simulink model "cn_i_128w_2k_do_al_r301"  (Simulink 6.2)
settings: Solver=ode45  StartTime=0.0  StopTime=1000  RelTol=1e-3
libraries: xbsIndex_r3 x390, xps_library x17, ddc_library x4, reorder_library x3, fft_library x2, pfb_library x2, simulink x1, delay_lib x1
(part 1 of 3)
settings Model: LastModifiedBy=manley
settings DebuggingCC: SolverPrmCheckMsg=warning

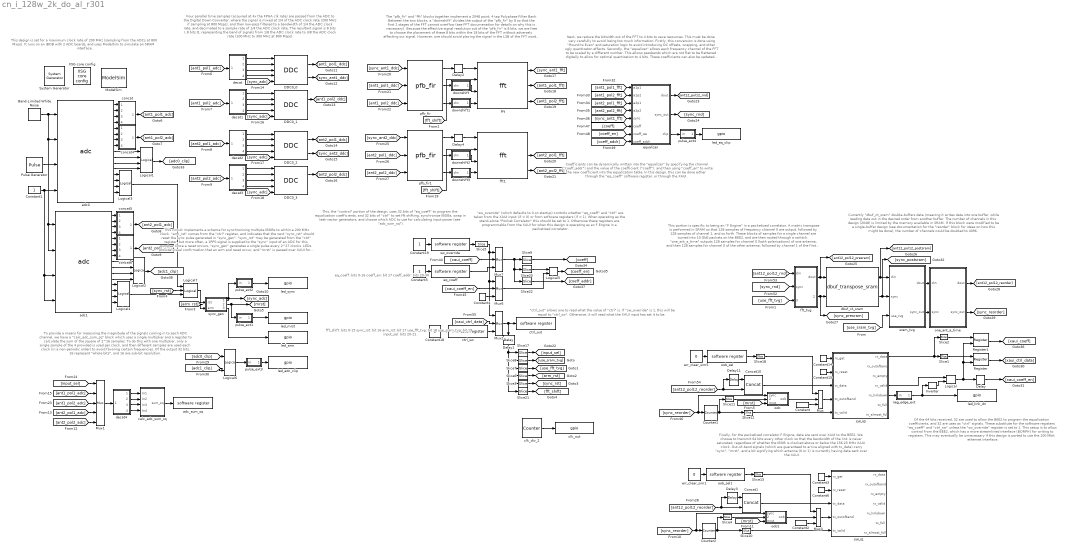
== system cn_i_128w_2k_do_al_r301 ==
  note: fft_shift: bits 0-15
      | sync_rst: bit 16
      | arm_rst: bit 17
      | use_fft_tvg: bit 18
      | use_sram_tvg: bit 19
      | input_sel: bits 20-21
  note: eq_coeff: bits 0-16
      | coeff_en: bit 17
      | coeff_addr: bits 20-30
  note: This design is set for a maximum
      | clock rate of 200 MHz (sampling
      | from the ADCs at 800 Mxps).  It
      | runs on an IBOB with 2 ADC boards,
      | and uses ModelSim to simulate an
      | SRAM interface.
  note: This circuit implements a scheme for synchronizing
      | multiple IBOBs to within a 200 MHz clock.  "arm_rst"
      | comes from the "ctrl" register, and indicates that the
      | next "sync_rst" should reset the sync pulse generated
      | in "sync_gen".  "sync_rst" may be generated from
      | the "ctrl" register, but more often, a 1PPS signal is
      | supplied to the "sync" input of an ADC for this
      | purpose.  Once a reset occurs, "sync_gen" generates
      | a single pulse every 2^27 clocks.  LEDs provide visual
      | confirmation that an arm and reset occur, and "mrst"
      | is passed over XAUI for the purpose of informing
      | downstream logic in a packetized correlator that
      | a "master reset" has occurred.
  note: "sw_override" (which defaults to 0 on startup)
      | controls whether "eq_coeff" and "ctrl" are taken
      | from the XAUI input (if = 0) or from software
      | registers (if = 1).  When operating as the stand-alone
      | "Pocket Correlator" this should be set to 1.  Otherwise
      | these registers are programmable from the XAUI for
      | when this design is operating as  an F Engine
      | in a packetized correlator.
  note: Four parallel time samples (acquired at 4x the
      | FPGA clk rate) are passed from the ADC to the
      | Digital Down Converter, where the signal is mixed
      | at 1/4 of the ADC clock rate (200 MHz if sampling
      | at 800 Msps), and then low-pass filtered to a
      | bandwidth of 1/4 the ADC clock rate, and decimated
      | to a sample rate of 1/4 the ADC clock rate.  The
      | resultant signal is 8 bits I, 8 bits Q, representing the
      | band of signals from 1/8 the ADC clock rate to
      | 3/8 the ADC clock rate (100 MHz to 300 MHz at
      | 800 Msps).
  note: The "pfb_fir" and "fft" blocks together implement a 2048 point,
      | 4 tap Polyphase Filter Bank.  Between the two blocks, a "downshift"
      | divides the output of the "pfb_fir" by 8 so that the first 2 stages of
      | the FFT cannot overflow (see FFT documenation for details on why
      | this is necessary).  Because the effective signal resolution out of
      | the "pfb_fir" is 8 bits, we are free to choose the placement of
      | these 8 bits within the 18 bits of the FFT without adversely affecting
      | our signal.  However, one should avoid placing the signal in the LSB
      | of the FFT word because of rounding effects.  Thus, we downshift
      | only 3 bits.
  note: Next, we reduce the bitwidth out of the FFT to 4 bits to save resources.
      | This must be done very carefully to avoid losing too much information.
      | Firstly, this conversion is done using "Round to Even" and saturation
      | logic to avoid introducing DC offsets, wrapping, and other ugly quantizaton
      | effects.  Secondly, the "equalizer" allows each frequency channel of the
      | FFT to be scaled by a different number.  This allows passbands which are
      | not flat to be flattened digitally to allow for optimal quantization to 4 bits.
      | These coefficients can also be updated dynamically for gain control.
  note: Coefficients can be dynamically written into the "equalizer" by
      | specifying the channel ("coeff_addr") and the value of the
      | coefficient ("coeff"), and then using "coeff_en" to write the
      | new coefficient into the equalization table.  In this design,
      | this can be done either through the "eq_coeff" software
      | register, or through the XAUI.
  note: To provide a means for measuring the magnitude of the signals
      | coming in to each ADC channel, we have a "calc_adc_sum_sq"
      | block which uses a single multiplier and a regsiter to calculate
      | the sum of the square of 2^16 samples.  To do this with one
      | multiplier, only a single sample of the 4 provided is used
      | per clock, and then different samples are used each clock (in
      | a non-periodic order) to avoid favoring certain frequencies.
      | Of the output 32 bits, 16 represent "whole bits", and 16
      | are sub-bit resolution.
  note: This portion is specific to being an "F Engine" in a packetized correlator.
      | A matrix transpose is performed in SRAM so that 128 samples of frequency
      | channel 0 are output, followed by 128 samples of channel 1, and so forth.
      | These blocks of samples for a single channel are turned into 10 GbE packets
      | on the BEE2, and are then routed through a swittch.  "one_ant_a_time"
      | outputs 128 samples for channel 0 (both polarizations) of one antenna,
      | and then 128 samples for channel 0 of the other antenna, followed by
      | channel 1 of the first antenna, and so on.  This allows the BEE2 design to
      | pass data directly from the XAUI into a packet containing 128 time samples
      | for 1 frequency from 1 antenna.
  note: Currently "dbuf_ct_sram" double-buffers data (meaning it writes data
      | into one buffer, while reading data out in the desired order from another
      | buffer.  The number of channels in this design (2048) is limited by the
      | memory available in SRAM.  If this block were modified to be a
      | single-buffer design (see documentation for the "reorder" block for
      | ideas on how this might be done), the number of channels could
      | be doubled to 4096.
  note: Finally, for the packetized correlator F Engine, data are sent over
      | XAUI to the BEE2.  We choose to transmit 64 bits every other clock
      | so that the bandwidth of the link is never saturated, regardless of whether
      | the IBOB is clocked above or below the 156.25 MHz XAUI clock.
      | Out-of-band signals (which are guaranteed to arrive aligned with
      | tx_data) carry "sync", "mrst", and a bit signifying which antenna (0 or 1)
      | is currently having data sent over the XAUI.
  note: Of the 64 bits received, 32 are used to allow the BEE2
      | to program the equalization coefficients, and 32 are
      | uses as "ctrl" signals.  These substitute for the software
      | registers "eq_coeff" and "ctrl_sw" unless the "sw_override"
      | register is set to 1.  This setup is to allow control from the
      | BEE2, which has a more streamlined interface (BORPH)
      | for writing to registers.  This may eventually be unnecessary
      | if this design is ported to use the 100 Mbit ethernet interface.
  note: This, the "control" portion of the design, uses
      | 32 bits of "eq_coeff" to program the equalization
      | coefficients, and 32 bits of "ctrl" to set fft shifting,
      | synchronize IBOBs, swap in test-vector generators,
      | and choose which ADC to use for calculating
      | input power (see "adc_sum_sq").
  note: "ctrl_out" allows one to read what the
      | value of "ctrl" is.  If "sw_override" is
      | 1, this will be equal to "ctrl_sw".  Otherwise,
      | it will read what the XAUI input has set
      | it to be.
  " System Generator" : xbsIndex_r3/ System Generator  Tag=genX  xilinxfamily=Virtex2P  part=xc2vp50  speed=-7  package=ff1152  synthesis_tool=XST  directory=./cn_i_128w_2k_x_rev3_astro_lib/sysgen  testbench=off  simulink_period=1  sysclk_period=5  incr_netlist=off  trim_vbits=Everywhere in SubSystem  dbl_ovrd=According to Block Masks  core_generation=According to Block Masks  run_coregen=off  deprecated_control=off  eval_field=0
      settings: AttributesFormatString=System\nGenerator
  Band-Limited White Noise : simulink/Sources/Band-Limited White Noise  Cov=[0.1]  Ts=0.1  seed=[23341]
  Concat1 : xbsIndex_r3/Concat  num_inputs=2  explicit_period=off  period=1  dbl_ovrd=off
  Concat10 : xbsIndex_r3/Concat  num_inputs=2  explicit_period=off  period=1  dbl_ovrd=off
  Constant : xbsIndex_r3/Constant  const=0  equ=P=C  arith_type=Unsigned  n_bits=8  bin_pt=0  opselect=C  inp2=PCIN>>17  opr=+  inp1=P  carry=CIN  iostate=0  explicit_period=off  period=1  dbl_ovrd=off
  Constant1 : Constant
  Constant14 : xbsIndex_r3/Constant  const=1  equ=P=C  arith_type=Unsigned  n_bits=1  bin_pt=0  opselect=C  inp2=PCIN>>17  opr=+  inp1=P  carry=CIN  iostate=0  explicit_period=on  period=1  dbl_ovrd=off
  Constant15 : xbsIndex_r3/Constant  const=0  equ=P=C  arith_type=Unsigned  n_bits=1  bin_pt=0  opselect=C  inp2=PCIN>>17  opr=+  inp1=P  carry=CIN  iostate=0  explicit_period=on  period=1  dbl_ovrd=off
  Constant18 : Constant  Value=0
  Constant19 : Constant
  Constant2 : xbsIndex_r3/Constant  const=0  equ=P=C  arith_type=Unsigned  n_bits=8  bin_pt=0  opselect=C  inp2=PCIN>>17  opr=+  inp1=P  carry=CIN  iostate=0  explicit_period=off  period=1  dbl_ovrd=off
  Constant3 : xbsIndex_r3/Constant  const=1  equ=P=C  arith_type=Unsigned  n_bits=1  bin_pt=0  opselect=C  inp2=PCIN>>17  opr=+  inp1=P  carry=CIN  iostate=0  explicit_period=on  period=1  dbl_ovrd=off
  Constant4 : xbsIndex_r3/Constant  const=1  equ=P=C  arith_type=Boolean  n_bits=1  bin_pt=0  opselect=C  inp2=PCIN>>17  opr=+  inp1=P  carry=CIN  iostate=0  explicit_period=on  period=1  dbl_ovrd=off
  Constant5 : Constant
  Constant6 : xbsIndex_r3/Constant  const=0  equ=P=C  arith_type=Unsigned  n_bits=1  bin_pt=0  opselect=C  inp2=PCIN>>17  opr=+  inp1=P  carry=CIN  iostate=0  explicit_period=on  period=1  dbl_ovrd=off
  Counter1 : xbsIndex_r3/Counter  cnt_type=Free Running  n_bits=7  bin_pt=0  arith_type=Unsigned  start_count=0  cnt_to=Inf  cnt_by_val=1  operation=Up  explicit_period=off  period=1  load_pin=off  rst=on  en=off  dbl_ovrd=off  show_param=off  use_rpm=on  gen_core=off
      settings: xl_area=[0, 0, 0, 0, 0, 0, 0]
  Counter2 : xbsIndex_r3/Counter  cnt_type=Free Running  n_bits=7  bin_pt=0  arith_type=Unsigned  start_count=0  cnt_to=Inf  cnt_by_val=1  operation=Up  explicit_period=off  period=1  load_pin=off  rst=on  en=off  dbl_ovrd=off  show_param=off  use_rpm=on  gen_core=off
      settings: xl_area=[0, 0, 0, 0, 0, 0, 0]
  DDC0_{0..3} (4 alike) : ddc_library/DDC  freq_div=4  lo_freq=1  num_inputs=4  lo_bitwidth=8  lpfir_coeff=".9 * [-0.0161   -0.0428   -0.0504   -0.0249    0.0354    0.1170    0.1948    0.2422    0.2422    0.1948    0.1170  0.0354   -0.0249   -0.0504   -0.0428   -0.0161]"  BitWidthOut=8  quantization="Round  (unbiased: Even Values)"  add_latency=1  mult_latency=2
  Delay : xbsIndex_r3/Delay  latency=1  reg_retiming=off  explicit_period=off  period=1  en=off  accept_only_valid=off  init_zero=on  dbl_ovrd=off  show_param=off
      settings: xl_area=[0, 0, 0, 0, 0, 0, 0]
  Delay1 : xbsIndex_r3/Delay  Orientation=down  latency=1  reg_retiming=off  explicit_period=off  period=1  en=off  accept_only_valid=off  init_zero=on  dbl_ovrd=off  show_param=off
      settings: xl_area=[0, 0, 0, 0, 0, 0, 0]
  Delay11 : xbsIndex_r3/Delay  latency=1  reg_retiming=off  explicit_period=off  period=1  en=off  accept_only_valid=off  init_zero=on  dbl_ovrd=off  show_param=off
      settings: xl_area=[0, 0, 0, 0, 0, 0, 0]
  Delay2 : xbsIndex_r3/Delay  latency=2  reg_retiming=off  explicit_period=off  period=1  en=off  accept_only_valid=off  init_zero=on  dbl_ovrd=off  show_param=off
      settings: xl_area=[0, 0, 0, 0, 0, 0, 0]
  Delay3 : xbsIndex_r3/Delay  latency=1  reg_retiming=off  explicit_period=off  period=1  en=off  accept_only_valid=off  init_zero=on  dbl_ovrd=off  show_param=off
      settings: xl_area=[0, 0, 0, 0, 0, 0, 0]
  Delay4 : xbsIndex_r3/Delay  latency=2  reg_retiming=off  explicit_period=off  period=1  en=off  accept_only_valid=off  init_zero=on  dbl_ovrd=off  show_param=off
      settings: xl_area=[0, 0, 0, 0, 0, 0, 0]
  Inverter : xbsIndex_r3/Inverter  latency=0  explicit_period=off  period=1  en=off  dbl_ovrd=off  show_param=off
      settings: xl_area=[0, 0, 0, 0, 0, 0, 0]
  Logical : xbsIndex_r3/Logical  logical_function=AND  inputs=2  precision=Full  arith_type=Unsigned  n_bits=8  bin_pt=2  align_bp=on  latency=0  explicit_period=off  period=1  en=off  dbl_ovrd=off  show_param=off
      settings: xl_area=[0, 0, 0, 0, 0, 0, 0]
  Logical{1..4} (4 alike) : xbsIndex_r3/Logical  logical_function=OR  inputs=4  precision=Full  arith_type=Unsigned  n_bits=8  bin_pt=2  align_bp=on  latency=1  explicit_period=off  period=1  en=off  dbl_ovrd=off  show_param=off
      settings: xl_area=[0, 0, 0, 0, 0, 0, 0]
  Logical5 : xbsIndex_r3/Logical  logical_function=AND  inputs=2  precision=Full  arith_type=Unsigned  n_bits=8  bin_pt=2  align_bp=on  latency=0  explicit_period=off  period=1  en=off  dbl_ovrd=off  show_param=off
      settings: xl_area=[0, 0, 0, 0, 0, 0, 0]
  Logical6 : xbsIndex_r3/Logical  logical_function=OR  inputs=2  precision=Full  arith_type=Unsigned  n_bits=8  bin_pt=2  align_bp=on  latency=1  explicit_period=off  period=1  en=off  dbl_ovrd=off  show_param=off
      settings: xl_area=[0, 0, 0, 0, 0, 0, 0]
  Logical7 : xbsIndex_r3/Logical  logical_function=OR  inputs=3  precision=Full  arith_type=Unsigned  n_bits=8  bin_pt=2  align_bp=on  latency=1  explicit_period=off  period=1  en=off  dbl_ovrd=off  show_param=off
      settings: xl_area=[0, 0, 0, 0, 0, 0, 0]
  ModelSim : xbsIndex_r3/ModelSim  dir=./modelsim  waveform=on  leave_open=on  skip_compile=off  custom_scripts=off  startup_timeout=40
  Mux : xbsIndex_r3/Mux  inputs=2  precision=Full  arith_type="Signed  (2's comp)"  n_bits=8  bin_pt=2  quantization=Truncate  overflow=Wrap  latency=0  explicit_period=off  period=1  en=off  dbl_ovrd=off  show_param=off  mux_type=off  use_rpm=off  gen_core=off
      settings: xl_area=[0, 0, 0, 0, 0, 0, 0]
  Mux1 : xbsIndex_r3/Mux  inputs=4  precision=Full  arith_type="Signed  (2's comp)"  n_bits=8  bin_pt=2  quantization=Truncate  overflow=Wrap  latency=2  explicit_period=on  period=1  en=off  dbl_ovrd=off  show_param=off  mux_type=off  use_rpm=off  gen_core=off
      settings: xl_area=[0, 0, 0, 0, 0, 0, 0]
  Mux2 : xbsIndex_r3/Mux  inputs=2  precision=Full  arith_type="Signed  (2's comp)"  n_bits=8  bin_pt=2  quantization=Truncate  overflow=Wrap  latency=1  explicit_period=on  period=1  en=off  dbl_ovrd=off  show_param=off  mux_type=off  use_rpm=off  gen_core=off
      settings: xl_area=[0, 0, 0, 0, 0, 0, 0]
  Mux3 : xbsIndex_r3/Mux  inputs=2  precision=Full  arith_type="Signed  (2's comp)"  n_bits=8  bin_pt=2  quantization=Truncate  overflow=Wrap  latency=0  explicit_period=off  period=1  en=off  dbl_ovrd=off  show_param=off  mux_type=off  use_rpm=off  gen_core=off
      settings: xl_area=[0, 0, 0, 0, 0, 0, 0]
  Mux6 : xbsIndex_r3/Mux  inputs=2  precision=Full  arith_type="Signed  (2's comp)"  n_bits=8  bin_pt=2  quantization=Truncate  overflow=Wrap  latency=1  explicit_period=on  period=1  en=off  dbl_ovrd=off  show_param=off  mux_type=off  use_rpm=off  gen_core=off
      settings: xl_area=[0, 0, 0, 0, 0, 0, 0]
  Mux7 : xbsIndex_r3/Mux  inputs=2  precision=Full  arith_type="Signed  (2's comp)"  n_bits=8  bin_pt=2  quantization=Truncate  overflow=Wrap  latency=1  explicit_period=on  period=1  en=off  dbl_ovrd=off  show_param=off  mux_type=off  use_rpm=off  gen_core=off
      settings: xl_area=[0, 0, 0, 0, 0, 0, 0]
  Pulse Generator : DiscretePulseGenerator  Period=2^27
  Register : xbsIndex_r3/Register  init=0  reg_only_valid=off  explicit_period=off  period=1  rst=off  en=on  out_en=off  dbl_ovrd=off  show_param=off
      settings: xl_area=[0, 0, 0, 0, 0, 0, 0]
  Register1 : xbsIndex_r3/Register  init=0  reg_only_valid=off  explicit_period=off  period=1  rst=off  en=on  out_en=off  dbl_ovrd=off  show_param=off
      settings: xl_area=[0, 0, 0, 0, 0, 0, 0]
  Slice1 : xbsIndex_r3/Slice  mode=Lower Bit Location + Width  nbits=32  bit1=0  base1=MSB of Input  bit0=0  base0=LSB of Input  boolean_output=on  explicit_period=off  period=1  dbl_ovrd=off
  Slice10 : xbsIndex_r3/Slice  mode=Lower Bit Location + Width  nbits=1  bit1=0  base1=MSB of Input  bit0=0  base0=LSB of Input  boolean_output=on  explicit_period=off  period=1  dbl_ovrd=off
  Slice11 : xbsIndex_r3/Slice  mode=Upper Bit Location + Width  nbits=1  bit1=0  base1=MSB of Input  bit0=0  base0=LSB of Input  boolean_output=on  explicit_period=off  period=1  dbl_ovrd=off
  Slice12 : xbsIndex_r3/Slice  mode=Lower Bit Location + Width  nbits=1  bit1=0  base1=MSB of Input  bit0=0  base0=LSB of Input  boolean_output=on  explicit_period=off  period=1  dbl_ovrd=off
  Slice13 : xbsIndex_r3/Slice  mode=Lower Bit Location + Width  nbits=1  bit1=0  base1=MSB of Input  bit0=0  base0=LSB of Input  boolean_output=off  explicit_period=off  period=1  dbl_ovrd=off
  Slice17 : xbsIndex_r3/Slice  mode=Lower Bit Location + Width  nbits=2  bit1=0  base1=MSB of Input  bit0=20  base0=LSB of Input  boolean_output=off  explicit_period=off  period=1  dbl_ovrd=off
  Slice18 : xbsIndex_r3/Slice  mode=Lower Bit Location + Width  nbits=1  bit1=0  base1=MSB of Input  bit0=0  base0=LSB of Input  boolean_output=off  explicit_period=off  period=1  dbl_ovrd=off
  Slice2 : xbsIndex_r3/Slice  mode=Lower Bit Location + Width  nbits=32  bit1=0  base1=MSB of Input  bit0=32  base0=LSB of Input  boolean_output=off  explicit_period=off  period=1  dbl_ovrd=off
  Slice20 : xbsIndex_r3/Slice  mode=Lower Bit Location + Width  nbits=1  bit1=0  base1=MSB of Input  bit0=17  base0=LSB of Input  boolean_output=on  explicit_period=off  period=1  dbl_ovrd=off
  Slice21 : xbsIndex_r3/Slice  mode=Lower Bit Location + Width  nbits=16  bit1=0  base1=MSB of Input  bit0=0  base0=LSB of Input  boolean_output=off  explicit_period=off  period=1  dbl_ovrd=off
  Slice22 : xbsIndex_r3/Slice  mode=Lower Bit Location + Width  nbits=11  bit1=0  base1=MSB of Input  bit0=20  base0=LSB of Input  boolean_output=off  explicit_period=off  period=1  dbl_ovrd=off
  Slice3 : xbsIndex_r3/Slice  mode=Lower Bit Location + Width  nbits=1  bit1=0  base1=MSB of Input  bit0=16  base0=LSB of Input  boolean_output=on  explicit_period=off  period=1  dbl_ovrd=off
  Slice4 : xbsIndex_r3/Slice  mode=Upper Bit Location + Width  nbits=1  bit1=0  base1=MSB of Input  bit0=0  base0=LSB of Input  boolean_output=on  explicit_period=off  period=1  dbl_ovrd=off
  Slice5 : xbsIndex_r3/Slice  mode=Lower Bit Location + Width  nbits=1  bit1=0  base1=MSB of Input  bit0=0  base0=LSB of Input  boolean_output=off  explicit_period=off  period=1  dbl_ovrd=off
  Slice6 : xbsIndex_r3/Slice  mode=Lower Bit Location + Width  nbits=1  bit1=0  base1=MSB of Input  bit0=17  base0=LSB of Input  boolean_output=on  explicit_period=off  period=1  dbl_ovrd=off
  Slice7 : xbsIndex_r3/Slice  mode=Lower Bit Location + Width  nbits=1  bit1=0  base1=MSB of Input  bit0=18  base0=LSB of Input  boolean_output=off  explicit_period=off  period=1  dbl_ovrd=off
  Slice8 : xbsIndex_r3/Slice  mode=Lower Bit Location + Width  nbits=1  bit1=0  base1=MSB of Input  bit0=19  base0=LSB of Input  boolean_output=off  explicit_period=off  period=1  dbl_ovrd=off
  Slice9 : xbsIndex_r3/Slice  mode=Lower Bit Location + Width  nbits=17  bit1=0  base1=MSB of Input  bit0=0  base0=LSB of Input  boolean_output=off  explicit_period=off  period=1  dbl_ovrd=off
  XAUI0 : Subsystem  Tag=xps:xaui  AncestorBlock=xps_library/XAUI  mask{demux=1, port=iBOB:0, show_param=off, pre_emph=3, swing=800}
      mask prompts: show_param "---------------------- Show Implementation Parameters -----------------------------------------------------------------------------------"; pre_emph "Pre-emphasis"; swing "Differential swing"
      mask init:
      | xaui_mask;
      mask StyleString: popup(1|2),popup(iBOB:0|iBOB:1|BEE2_ctrl:0|BEE2_ctrl:1|BEE2_usr:0|BEE2_usr:1|BEE2_usr:2|BEE2_usr:3|CORR:0),checkbox,popup(0|1|2|3),popup(400|500|600|700|800)
      mask CallbackString:
      | ||myname=gcb;
      | if strcmp(get_param(myname, 'show_param'), 'on')
      |     set_param(myname, 'MaskVisibilities', {'on','on','on','on','on'});
      | else
      |     set_param(myname, 'MaskVisibilities', {'on','on','on','off','off'});
      | end||
  XAUI1 : Subsystem  Tag=xps:xaui  AncestorBlock=xps_library/XAUI  mask{demux=1, port=iBOB:1, show_param=off, pre_emph=3, swing=800}
      mask prompts: show_param "---------------------- Show Implementation Parameters -----------------------------------------------------------------------------------"; pre_emph "Pre-emphasis"; swing "Differential swing"
      mask init:
      | xaui_mask;
      mask StyleString: popup(1|2),popup(iBOB:0|iBOB:1|BEE2_ctrl:0|BEE2_ctrl:1|BEE2_usr:0|BEE2_usr:1|BEE2_usr:2|BEE2_usr:3|CORR:0),checkbox,popup(0|1|2|3),popup(400|500|600|700|800)
      mask CallbackString:
      | ||myname=gcb;
      | if strcmp(get_param(myname, 'show_param'), 'on')
      |     set_param(myname, 'MaskVisibilities', {'on','on','on','on','on'});
      | else
      |     set_param(myname, 'MaskVisibilities', {'on','on','on','off','off'});
      | end||
  XSG core config : xps_library/XSG core config  Tag=xps:xsg  hw_sys=iBOB  ibob_linux=off  clk_src=adc0_clk  gpio_clk_io_group=iBOB:sma  gpio_clk_bit_index=0  clk_rate=200  sample_period=1  synthesis_tool=XST  mpc_type=powerpc405
  adc0 : xps_library/adc  Tag=xps:adc  adc_brd=iBOB:adc0  adc_clk_rate=600  adc_interleave=off  sample_period=1
  adc1 : xps_library/adc  Tag=xps:adc  adc_brd=iBOB:adc1  adc_clk_rate=600  adc_interleave=off  sample_period=1
  adc_sum_sq : xps_library/software register  Tag=xps:sw_reg  io_dir=To Processor  arith_type=Unsigned  bitwidth=32  bin_pt=14  sample_period=1  gw_name=cn_i_128w_2k_dualout_al_adc_sum_sq_user_data_in
  calc_adc_sum_sq : Subsystem
  clk_div_2 : xbsIndex_r3/Counter  cnt_type=Free Running  n_bits=1  bin_pt=0  arith_type=Unsigned  start_count=0  cnt_to=Inf  cnt_by_val=1  operation=Up  explicit_period=off  period=1  load_pin=off  rst=off  en=off  dbl_ovrd=off  show_param=off  use_rpm=on  gen_core=off
      settings: xl_area=[0, 0, 0, 0, 0, 0, 0]
  clk_out : xps_library/gpio  Tag=xps:gpio  io_group=iBOB:sma  io_dir=out  arith_type=Unsigned  bitwidth=1  bin_pt=0  bit_index=0  sample_period=1  use_ddr=off  reg_iob=on  reg_clk_phase=0  termination=None
  concat : Subsystem
  concat4 : Subsystem
  concat5 : Subsystem
  concat6 : Subsystem
  ctrl_out : xps_library/software register  Tag=xps:sw_reg  io_dir=To Processor  arith_type=Unsigned  bitwidth=32  bin_pt=0  sample_period=1  gw_name=cn_i_128w_2k_dualout_al_ctrl_out_user_data_in
  ctrl_sw : xps_library/software register  Tag=xps:sw_reg  io_dir=From Processor  arith_type=Unsigned  bitwidth=32  bin_pt=0  sample_period=1  gw_name=cn_i_128w_2k_dualout_al_ctrl_sw_user_data_out
  dbuf_ct_sram : reorder_library/dbuf_transpose_sram  length=2^11  numSpecs=128
      link override sync_delay/Constant: equ=P=C
      link override sync_delay/Constant1: equ=P=C
      link override sync_delay/Constant2: equ=P=C
      link override sync_delay/Constant3: equ=P=C
  decat : Subsystem
  decat1 : Subsystem
  decat2 : Subsystem
  decat3 : Subsystem
  decat4 : Subsystem
  downshift : Subsystem
  downshift1 : Subsystem
  downshift2 : Subsystem
  downshift3 : Subsystem
  eq_coeff : xps_library/software register  Tag=xps:sw_reg  io_dir=From Processor  arith_type=Unsigned  bitwidth=32  bin_pt=0  sample_period=1  gw_name=cn_i_128w_2k_dualout_al_eq_coeff_user_data_out
  equalizer : Subsystem
  err_clear_sim1 : Constant  Value=0
  err_clear_sim5 : Constant  Value=0
  fft : fft_library/fft  FFTSize=11  BitWidth=18  n_inputs=0  quantization="Round  (unbiased: Even Values)"  overflow=Wrap  add_latency=1  mult_latency=2  bram_latency=2
  fft1 : fft_library/fft  FFTSize=11  BitWidth=18  n_inputs=0  quantization="Round  (unbiased: Even Values)"  overflow=Wrap  add_latency=1  mult_latency=2  bram_latency=2
  fft_tvg : Subsystem
  led_adc_clip : xps_library/gpio  Tag=xps:gpio  io_group=iBOB:led  io_dir=out  arith_type=Boolean  bitwidth=1  bin_pt=0  bit_index=5  sample_period=1  use_ddr=off  reg_iob=on  reg_clk_phase=0  termination=None
  led_arm : xps_library/gpio  Tag=xps:gpio  io_group=iBOB:led  io_dir=out  arith_type=Boolean  bitwidth=1  bin_pt=0  bit_index=0  sample_period=1  use_ddr=off  reg_iob=on  reg_clk_phase=0  termination=None
  led_eq_clip : xps_library/gpio  Tag=xps:gpio  io_group=iBOB:led  io_dir=out  arith_type=Boolean  bitwidth=1  bin_pt=0  bit_index=7  sample_period=1  use_ddr=off  reg_iob=on  reg_clk_phase=0  termination=None
  led_link_dn : xps_library/gpio  Tag=xps:gpio  io_group=iBOB:led  io_dir=out  arith_type=Unsigned  bitwidth=1  bin_pt=0  bit_index=6  sample_period=1  use_ddr=off  reg_iob=on  reg_clk_phase=0  termination=None
  led_mrst : xps_library/gpio  Tag=xps:gpio  io_group=iBOB:led  io_dir=out  arith_type=Boolean  bitwidth=1  bin_pt=0  bit_index=3  sample_period=1  use_ddr=off  reg_iob=on  reg_clk_phase=0  termination=None
  led_sync : xps_library/gpio  Tag=xps:gpio  io_group=iBOB:led  io_dir=out  arith_type=Boolean  bitwidth=1  bin_pt=0  bit_index=2  sample_period=1  use_ddr=off  reg_iob=on  reg_clk_phase=0  termination=None
  neg_edge_ext : Subsystem  mask{pulse_len=2^27}
      mask prompts: pulse_len "Length of Pulse"
      mask init:
      | bits = ceil(log2(pulse_len+1));
  one_ant_a_time : Subsystem
  oob : Subsystem
  oob1 : Subsystem
  oob_sel : xps_library/software register  Tag=xps:sw_reg  io_dir=From Processor  arith_type=Unsigned  bitwidth=32  bin_pt=0  sample_period=1  gw_name=cn_i_128w_2k_dualout_al_oob_sel_user_data_out
  oob_sel1 : xps_library/software register  Tag=xps:sw_reg  io_dir=From Processor  arith_type=Unsigned  bitwidth=32  bin_pt=0  sample_period=1  gw_name=cn_i_128w_2k_dualout_al_oob_sel1_user_data_out
  pfb_fir : pfb_library/pfb_fir  PFBSize=11  TotalTaps=4  WindowType=hamming  n_inputs=0  MakeBiplex=on  BitWidthIn=8  BitWidthOut=18  CoeffBitWidth=8  CoeffDistMem=off  add_latency=1  mult_latency=2  bram_latency=2  quantization="Round  (unbiased: Even Values)"  fwidth=1
      link override pol1_in1_first_tap/sync_delay/Constant: equ=P=C
      link override pol1_in1_first_tap/sync_delay/Constant1: equ=P=C
      link override pol1_in1_first_tap/sync_delay/Constant2: equ=P=C
      link override pol1_in1_first_tap/sync_delay/Constant3: equ=P=C
      link override pol1_in1_tap10/sync_delay/Constant: equ=P=C
      link override pol1_in1_tap10/sync_delay/Constant1: equ=P=C
      link override pol1_in1_tap10/sync_delay/Constant2: equ=P=C
      link override pol1_in1_tap10/sync_delay/Constant3: equ=P=C
      link override pol1_in1_tap11/sync_delay/Constant: equ=P=C
      link override pol1_in1_tap11/sync_delay/Constant1: equ=P=C
      link override pol1_in1_tap11/sync_delay/Constant2: equ=P=C
      link override pol1_in1_tap11/sync_delay/Constant3: equ=P=C
      link override pol1_in1_tap12/sync_delay/Constant: equ=P=C
      link override pol1_in1_tap12/sync_delay/Constant1: equ=P=C
      link override pol1_in1_tap12/sync_delay/Constant2: equ=P=C
      link override pol1_in1_tap12/sync_delay/Constant3: equ=P=C
      link override pol1_in1_tap13/sync_delay/Constant: equ=P=C
      link override pol1_in1_tap13/sync_delay/Constant1: equ=P=C
      link override pol1_in1_tap13/sync_delay/Constant2: equ=P=C
      link override pol1_in1_tap13/sync_delay/Constant3: equ=P=C
      link override pol1_in1_tap14/sync_delay/Constant: equ=P=C
      link override pol1_in1_tap14/sync_delay/Constant1: equ=P=C
      link override pol1_in1_tap14/sync_delay/Constant2: equ=P=C
      link override pol1_in1_tap14/sync_delay/Constant3: equ=P=C
      link override pol1_in1_tap15/sync_delay/Constant: equ=P=C
      link override pol1_in1_tap15/sync_delay/Constant1: equ=P=C
      link override pol1_in1_tap15/sync_delay/Constant2: equ=P=C
      link override pol1_in1_tap15/sync_delay/Constant3: equ=P=C
      link override pol1_in1_tap2/sync_delay/Constant: equ=P=C
      link override pol1_in1_tap2/sync_delay/Constant1: equ=P=C
      link override pol1_in1_tap2/sync_delay/Constant2: equ=P=C
      link override pol1_in1_tap2/sync_delay/Constant3: equ=P=C
      link override pol1_in1_tap3/sync_delay/Constant: equ=P=C
      link override pol1_in1_tap3/sync_delay/Constant1: equ=P=C
      link override pol1_in1_tap3/sync_delay/Constant2: equ=P=C
      link override pol1_in1_tap3/sync_delay/Constant3: equ=P=C
      link override pol1_in1_tap4/sync_delay/Constant: equ=P=C
      link override pol1_in1_tap4/sync_delay/Constant1: equ=P=C
      link override pol1_in1_tap4/sync_delay/Constant2: equ=P=C
      link override pol1_in1_tap4/sync_delay/Constant3: equ=P=C
      link override pol1_in1_tap5/sync_delay/Constant: equ=P=C
      link override pol1_in1_tap5/sync_delay/Constant1: equ=P=C
      link override pol1_in1_tap5/sync_delay/Constant2: equ=P=C
      link override pol1_in1_tap5/sync_delay/Constant3: equ=P=C
      link override pol1_in1_tap6/sync_delay/Constant: equ=P=C
      link override pol1_in1_tap6/sync_delay/Constant1: equ=P=C
      link override pol1_in1_tap6/sync_delay/Constant2: equ=P=C
      link override pol1_in1_tap6/sync_delay/Constant3: equ=P=C
      link override pol1_in1_tap7/sync_delay/Constant: equ=P=C
      link override pol1_in1_tap7/sync_delay/Constant1: equ=P=C
      link override pol1_in1_tap7/sync_delay/Constant2: equ=P=C
      link override pol1_in1_tap7/sync_delay/Constant3: equ=P=C
      link override pol1_in1_tap8/sync_delay/Constant: equ=P=C
      link override pol1_in1_tap8/sync_delay/Constant1: equ=P=C
      link override pol1_in1_tap8/sync_delay/Constant2: equ=P=C
      link override pol1_in1_tap8/sync_delay/Constant3: equ=P=C
      link override pol1_in1_tap9/sync_delay/Constant: equ=P=C
      link override pol1_in1_tap9/sync_delay/Constant1: equ=P=C
      link override pol1_in1_tap9/sync_delay/Constant2: equ=P=C
      link override pol1_in1_tap9/sync_delay/Constant3: equ=P=C
      link override pol2_in1_first_tap/sync_delay/Constant: equ=P=C
      link override pol2_in1_first_tap/sync_delay/Constant1: equ=P=C
      link override pol2_in1_first_tap/sync_delay/Constant2: equ=P=C
      link override pol2_in1_first_tap/sync_delay/Constant3: equ=P=C
      link override pol2_in1_tap10/sync_delay/Constant: equ=P=C
      link override pol2_in1_tap10/sync_delay/Constant1: equ=P=C
      link override pol2_in1_tap10/sync_delay/Constant2: equ=P=C
      link override pol2_in1_tap10/sync_delay/Constant3: equ=P=C
      link override pol2_in1_tap11/sync_delay/Constant: equ=P=C
      link override pol2_in1_tap11/sync_delay/Constant1: equ=P=C
      link override pol2_in1_tap11/sync_delay/Constant2: equ=P=C
      link override pol2_in1_tap11/sync_delay/Constant3: equ=P=C
      link override pol2_in1_tap12/sync_delay/Constant: equ=P=C
      link override pol2_in1_tap12/sync_delay/Constant1: equ=P=C
      link override pol2_in1_tap12/sync_delay/Constant2: equ=P=C
      link override pol2_in1_tap12/sync_delay/Constant3: equ=P=C
      link override pol2_in1_tap13/sync_delay/Constant: equ=P=C
      link override pol2_in1_tap13/sync_delay/Constant1: equ=P=C
      link override pol2_in1_tap13/sync_delay/Constant2: equ=P=C
      link override pol2_in1_tap13/sync_delay/Constant3: equ=P=C
      link override pol2_in1_tap14/sync_delay/Constant: equ=P=C
      link override pol2_in1_tap14/sync_delay/Constant1: equ=P=C
      link override pol2_in1_tap14/sync_delay/Constant2: equ=P=C
      link override pol2_in1_tap14/sync_delay/Constant3: equ=P=C
      link override pol2_in1_tap15/sync_delay/Constant: equ=P=C
      link override pol2_in1_tap15/sync_delay/Constant1: equ=P=C
      link override pol2_in1_tap15/sync_delay/Constant2: equ=P=C
      link override pol2_in1_tap15/sync_delay/Constant3: equ=P=C
      link override pol2_in1_tap2/sync_delay/Constant: equ=P=C
      link override pol2_in1_tap2/sync_delay/Constant1: equ=P=C
      link override pol2_in1_tap2/sync_delay/Constant2: equ=P=C
      link override pol2_in1_tap2/sync_delay/Constant3: equ=P=C
      link override pol2_in1_tap3/sync_delay/Constant: equ=P=C
      link override pol2_in1_tap3/sync_delay/Constant1: equ=P=C
      link override pol2_in1_tap3/sync_delay/Constant2: equ=P=C
      link override pol2_in1_tap3/sync_delay/Constant3: equ=P=C
      link override pol2_in1_tap4/sync_delay/Constant: equ=P=C
      link override pol2_in1_tap4/sync_delay/Constant1: equ=P=C
      link override pol2_in1_tap4/sync_delay/Constant2: equ=P=C
      link override pol2_in1_tap4/sync_delay/Constant3: equ=P=C
      link override pol2_in1_tap5/sync_delay/Constant: equ=P=C
      link override pol2_in1_tap5/sync_delay/Constant1: equ=P=C
      link override pol2_in1_tap5/sync_delay/Constant2: equ=P=C
      link override pol2_in1_tap5/sync_delay/Constant3: equ=P=C
      link override pol2_in1_tap6/sync_delay/Constant: equ=P=C
      link override pol2_in1_tap6/sync_delay/Constant1: equ=P=C
      link override pol2_in1_tap6/sync_delay/Constant2: equ=P=C
      link override pol2_in1_tap6/sync_delay/Constant3: equ=P=C
      link override pol2_in1_tap7/sync_delay/Constant: equ=P=C
      link override pol2_in1_tap7/sync_delay/Constant1: equ=P=C
      link override pol2_in1_tap7/sync_delay/Constant2: equ=P=C
      link override pol2_in1_tap7/sync_delay/Constant3: equ=P=C
      link override pol2_in1_tap8/sync_delay/Constant: equ=P=C
      link override pol2_in1_tap8/sync_delay/Constant1: equ=P=C
      link override pol2_in1_tap8/sync_delay/Constant2: equ=P=C
      link override pol2_in1_tap8/sync_delay/Constant3: equ=P=C
      link override pol2_in1_tap9/sync_delay/Constant: equ=P=C
      link override pol2_in1_tap9/sync_delay/Constant1: equ=P=C
      link override pol2_in1_tap9/sync_delay/Constant2: equ=P=C
      link override pol2_in1_tap9/sync_delay/Constant3: equ=P=C
  pfb_fir1 : pfb_library/pfb_fir  PFBSize=11  TotalTaps=4  WindowType=hamming  n_inputs=0  MakeBiplex=on  BitWidthIn=8  BitWidthOut=18  CoeffBitWidth=8  CoeffDistMem=off  add_latency=1  mult_latency=2  bram_latency=2  quantization="Round  (unbiased: Even Values)"  fwidth=1
      link override pol1_in1_first_tap/sync_delay/Constant: equ=P=C
      link override pol1_in1_first_tap/sync_delay/Constant1: equ=P=C
      link override pol1_in1_first_tap/sync_delay/Constant2: equ=P=C
      link override pol1_in1_first_tap/sync_delay/Constant3: equ=P=C
      link override pol1_in1_tap10/sync_delay/Constant: equ=P=C
      link override pol1_in1_tap10/sync_delay/Constant1: equ=P=C
      link override pol1_in1_tap10/sync_delay/Constant2: equ=P=C
      link override pol1_in1_tap10/sync_delay/Constant3: equ=P=C
      link override pol1_in1_tap11/sync_delay/Constant: equ=P=C
      link override pol1_in1_tap11/sync_delay/Constant1: equ=P=C
      link override pol1_in1_tap11/sync_delay/Constant2: equ=P=C
      link override pol1_in1_tap11/sync_delay/Constant3: equ=P=C
      link override pol1_in1_tap12/sync_delay/Constant: equ=P=C
      link override pol1_in1_tap12/sync_delay/Constant1: equ=P=C
      link override pol1_in1_tap12/sync_delay/Constant2: equ=P=C
      link override pol1_in1_tap12/sync_delay/Constant3: equ=P=C
      link override pol1_in1_tap13/sync_delay/Constant: equ=P=C
      link override pol1_in1_tap13/sync_delay/Constant1: equ=P=C
      link override pol1_in1_tap13/sync_delay/Constant2: equ=P=C
      link override pol1_in1_tap13/sync_delay/Constant3: equ=P=C
      link override pol1_in1_tap14/sync_delay/Constant: equ=P=C
      link override pol1_in1_tap14/sync_delay/Constant1: equ=P=C
      link override pol1_in1_tap14/sync_delay/Constant2: equ=P=C
      link override pol1_in1_tap14/sync_delay/Constant3: equ=P=C
      link override pol1_in1_tap15/sync_delay/Constant: equ=P=C
      link override pol1_in1_tap15/sync_delay/Constant1: equ=P=C
      link override pol1_in1_tap15/sync_delay/Constant2: equ=P=C
      link override pol1_in1_tap15/sync_delay/Constant3: equ=P=C
      link override pol1_in1_tap2/sync_delay/Constant: equ=P=C
      link override pol1_in1_tap2/sync_delay/Constant1: equ=P=C
      link override pol1_in1_tap2/sync_delay/Constant2: equ=P=C
      link override pol1_in1_tap2/sync_delay/Constant3: equ=P=C
      link override pol1_in1_tap3/sync_delay/Constant: equ=P=C
      link override pol1_in1_tap3/sync_delay/Constant1: equ=P=C
      link override pol1_in1_tap3/sync_delay/Constant2: equ=P=C
      link override pol1_in1_tap3/sync_delay/Constant3: equ=P=C
      link override pol1_in1_tap4/sync_delay/Constant: equ=P=C
      link override pol1_in1_tap4/sync_delay/Constant1: equ=P=C
      link override pol1_in1_tap4/sync_delay/Constant2: equ=P=C
      link override pol1_in1_tap4/sync_delay/Constant3: equ=P=C
      link override pol1_in1_tap5/sync_delay/Constant: equ=P=C
      link override pol1_in1_tap5/sync_delay/Constant1: equ=P=C
      link override pol1_in1_tap5/sync_delay/Constant2: equ=P=C
      link override pol1_in1_tap5/sync_delay/Constant3: equ=P=C
      link override pol1_in1_tap6/sync_delay/Constant: equ=P=C
      link override pol1_in1_tap6/sync_delay/Constant1: equ=P=C
      link override pol1_in1_tap6/sync_delay/Constant2: equ=P=C
      link override pol1_in1_tap6/sync_delay/Constant3: equ=P=C
      link override pol1_in1_tap7/sync_delay/Constant: equ=P=C
      link override pol1_in1_tap7/sync_delay/Constant1: equ=P=C
      link override pol1_in1_tap7/sync_delay/Constant2: equ=P=C
      link override pol1_in1_tap7/sync_delay/Constant3: equ=P=C
      link override pol1_in1_tap8/sync_delay/Constant: equ=P=C
      link override pol1_in1_tap8/sync_delay/Constant1: equ=P=C
      link override pol1_in1_tap8/sync_delay/Constant2: equ=P=C
      link override pol1_in1_tap8/sync_delay/Constant3: equ=P=C
      link override pol1_in1_tap9/sync_delay/Constant: equ=P=C
      link override pol1_in1_tap9/sync_delay/Constant1: equ=P=C
      link override pol1_in1_tap9/sync_delay/Constant2: equ=P=C
      link override pol1_in1_tap9/sync_delay/Constant3: equ=P=C
      link override pol2_in1_first_tap/sync_delay/Constant: equ=P=C
      link override pol2_in1_first_tap/sync_delay/Constant1: equ=P=C
      link override pol2_in1_first_tap/sync_delay/Constant2: equ=P=C
      link override pol2_in1_first_tap/sync_delay/Constant3: equ=P=C
      link override pol2_in1_tap10/sync_delay/Constant: equ=P=C
      link override pol2_in1_tap10/sync_delay/Constant1: equ=P=C
      link override pol2_in1_tap10/sync_delay/Constant2: equ=P=C
      link override pol2_in1_tap10/sync_delay/Constant3: equ=P=C
      link override pol2_in1_tap11/sync_delay/Constant: equ=P=C
      link override pol2_in1_tap11/sync_delay/Constant1: equ=P=C
      link override pol2_in1_tap11/sync_delay/Constant2: equ=P=C
      link override pol2_in1_tap11/sync_delay/Constant3: equ=P=C
      link override pol2_in1_tap12/sync_delay/Constant: equ=P=C
      link override pol2_in1_tap12/sync_delay/Constant1: equ=P=C
      link override pol2_in1_tap12/sync_delay/Constant2: equ=P=C
      link override pol2_in1_tap12/sync_delay/Constant3: equ=P=C
      link override pol2_in1_tap13/sync_delay/Constant: equ=P=C
      link override pol2_in1_tap13/sync_delay/Constant1: equ=P=C
      link override pol2_in1_tap13/sync_delay/Constant2: equ=P=C
      link override pol2_in1_tap13/sync_delay/Constant3: equ=P=C
      link override pol2_in1_tap14/sync_delay/Constant: equ=P=C
      link override pol2_in1_tap14/sync_delay/Constant1: equ=P=C
      link override pol2_in1_tap14/sync_delay/Constant2: equ=P=C
      link override pol2_in1_tap14/sync_delay/Constant3: equ=P=C
      link override pol2_in1_tap15/sync_delay/Constant: equ=P=C
      link override pol2_in1_tap15/sync_delay/Constant1: equ=P=C
      link override pol2_in1_tap15/sync_delay/Constant2: equ=P=C
      link override pol2_in1_tap15/sync_delay/Constant3: equ=P=C
      link override pol2_in1_tap2/sync_delay/Constant: equ=P=C
      link override pol2_in1_tap2/sync_delay/Constant1: equ=P=C
      link override pol2_in1_tap2/sync_delay/Constant2: equ=P=C
      link override pol2_in1_tap2/sync_delay/Constant3: equ=P=C
      link override pol2_in1_tap3/sync_delay/Constant: equ=P=C
      link override pol2_in1_tap3/sync_delay/Constant1: equ=P=C
      link override pol2_in1_tap3/sync_delay/Constant2: equ=P=C
      link override pol2_in1_tap3/sync_delay/Constant3: equ=P=C
      link override pol2_in1_tap4/sync_delay/Constant: equ=P=C
      link override pol2_in1_tap4/sync_delay/Constant1: equ=P=C
      link override pol2_in1_tap4/sync_delay/Constant2: equ=P=C
      link override pol2_in1_tap4/sync_delay/Constant3: equ=P=C
      link override pol2_in1_tap5/sync_delay/Constant: equ=P=C
      link override pol2_in1_tap5/sync_delay/Constant1: equ=P=C
      link override pol2_in1_tap5/sync_delay/Constant2: equ=P=C
      link override pol2_in1_tap5/sync_delay/Constant3: equ=P=C
      link override pol2_in1_tap6/sync_delay/Constant: equ=P=C
      link override pol2_in1_tap6/sync_delay/Constant1: equ=P=C
      link override pol2_in1_tap6/sync_delay/Constant2: equ=P=C
      link override pol2_in1_tap6/sync_delay/Constant3: equ=P=C
      link override pol2_in1_tap7/sync_delay/Constant: equ=P=C
      link override pol2_in1_tap7/sync_delay/Constant1: equ=P=C
      link override pol2_in1_tap7/sync_delay/Constant2: equ=P=C
      link override pol2_in1_tap7/sync_delay/Constant3: equ=P=C
      link override pol2_in1_tap8/sync_delay/Constant: equ=P=C
      link override pol2_in1_tap8/sync_delay/Constant1: equ=P=C
      link override pol2_in1_tap8/sync_delay/Constant2: equ=P=C
      link override pol2_in1_tap8/sync_delay/Constant3: equ=P=C
      link override pol2_in1_tap9/sync_delay/Constant: equ=P=C
      link override pol2_in1_tap9/sync_delay/Constant1: equ=P=C
      link override pol2_in1_tap9/sync_delay/Constant2: equ=P=C
      link override pol2_in1_tap9/sync_delay/Constant3: equ=P=C
  pulse_ext1 : Subsystem  mask{pulse_len=2^23}
      mask prompts: pulse_len "Length of Pulse"
      mask init:
      | bits = ceil(log2(pulse_len+1));
  pulse_ext2 : Subsystem  mask{pulse_len=2^23}
      mask prompts: pulse_len "Length of Pulse"
      mask init:
      | bits = ceil(log2(pulse_len+1));
  pulse_ext3 : Subsystem  mask{pulse_len=2^23}
      mask prompts: pulse_len "Length of Pulse"
      mask init:
      | bits = ceil(log2(pulse_len+1));
  pulse_ext4 : Subsystem  mask{pulse_len=2^23}
      mask prompts: pulse_len "Length of Pulse"
      mask init:
      | bits = ceil(log2(pulse_len+1));
  sram_tvg : Subsystem
  sw_override : xps_library/software register  Tag=xps:sw_reg  io_dir=From Processor  arith_type=Unsigned  bitwidth=32  bin_pt=0  sample_period=1  gw_name=cn_i_128w_2k_dualout_al_sw_override_user_data_out
  sync_gen : Subsystem
  wires:
  Pulse Generator/1 -> adc0/3
  Constant1/1 -> adc0/4, adc1/4, adc1/3
  Band-Limited White Noise/1 -> adc0/1, adc0/2, adc1/1, adc1/2
  fft_tvg/1(dout) -> dbuf_ct_sram/1, [ant12_pol12_presram]
  dbuf_ct_sram/2 -> sram_tvg/2(sync), [sync_postsram]
  dbuf_ct_sram/1 -> sram_tvg/1(din), [ant12_pol12_postsram]
  pfb_fir/1 -> Delay2/1
  pfb_fir1/1 -> Delay4/1
  pulse_ext2/1(out) -> led_sync/1
  sync_gen/1(sync) -> [sync_adc], pulse_ext2/1(in)
  pulse_ext1/1(out) -> led_mrst/1
  sram_tvg/1(dout) -> one_ant_a_time/1(din)
  sram_tvg/2(sync_out) -> one_ant_a_time/2(sync)
  Constant14/1 -> XAUI0/1(rx_get)
  Constant15/1 -> XAUI0/2(rx_reset)
  XAUI0/5(rx_linkdown) -> neg_edge_ext/1(in)
  Delay11/1 -> Concat10/1
  Concat10/1 -> XAUI0/3(tx_data)
  Counter1/1 -> Slice12/1, Slice11/1
  Slice12/1 -> XAUI0/5(tx_valid)
  Slice11/1 -> oob/2(antbit)
  adc0/13 -> Logical3/1
  adc0/14 -> Logical3/2
  adc0/15 -> Logical3/3
  adc0/16 -> Logical3/4
  adc1/13 -> Logical4/1
  adc1/14 -> Logical4/2
  adc1/15 -> Logical4/3
  adc1/16 -> Logical4/4
  Logical3/1 -> Logical7/1
  Logical7/1 -> sync_gen/1(rst)
  sync_gen/2(mrst) -> pulse_ext1/1(in), [mrst]
  Constant18/1 -> ctrl_sw/1
  Constant19/1 -> sw_override/1
  sw_override/1 -> Slice5/1
  Slice5/1 -> Mux7/1, Mux6/1, Mux2/1
  Mux2/1 -> ctrl_out/1, Delay1/1
  ctrl_sw/1 -> Mux2/3
  Slice8/1 -> [use_sram_tvg]
  [use_sram_tvg] -> sram_tvg/3(use_tvg)
  Slice7/1 -> [use_fft_tvg]
  Slice6/1 -> [arm_rst]
  Slice3/1 -> [sync_rst]
  Slice21/1 -> [fft_shift]
  [use_fft_tvg] -> fft_tvg/3(use_tvg)
  [arm_rst] -> sync_gen/2(arm)
  [mrst] -> oob/3(mrst)
  decat/1(Out1) -> DDC0_0/1
  decat/2(Out2) -> DDC0_0/2
  decat/3(Out3) -> DDC0_0/3
  decat/4(Out4) -> DDC0_0/4
  adc0/1 -> concat/1(In1)
  adc0/2 -> concat/2(In2)
  adc0/3 -> concat/3(In3)
  adc0/4 -> concat/4(In4)
  concat/1(Out1) -> [ant1_pol1_adc]
  [ant1_pol1_adc] -> decat/1(In1)
  concat4/1(Out1) -> [ant1_pol2_adc]
  adc0/5 -> concat4/1(In1)
  adc0/6 -> concat4/2(In2)
  adc0/7 -> concat4/3(In3)
  adc0/8 -> concat4/4(In4)
  concat5/1(Out1) -> [ant2_pol1_adc]
  concat6/1(Out1) -> [ant2_pol2_adc]
  adc1/1 -> concat5/1(In1)
  adc1/2 -> concat5/2(In2)
  adc1/3 -> concat5/3(In3)
  adc1/4 -> concat5/4(In4)
  adc1/5 -> concat6/1(In1)
  adc1/6 -> concat6/2(In2)
  adc1/7 -> concat6/3(In3)
  adc1/8 -> concat6/4(In4)
  [sync_rst] -> Logical7/2
  Logical4/1 -> Logical7/3
  [ant1_pol2_adc] -> decat1/1(In1)
  decat1/1(Out1) -> DDC0_1/1
  decat1/2(Out2) -> DDC0_1/2
  decat1/3(Out3) -> DDC0_1/3
  decat1/4(Out4) -> DDC0_1/4
  [ant2_pol1_adc] -> decat2/1(In1)
  [ant2_pol2_adc] -> decat3/1(In1)
  decat2/1(Out1) -> DDC0_2/1
  decat2/2(Out2) -> DDC0_2/2
  decat2/3(Out3) -> DDC0_2/3
  decat2/4(Out4) -> DDC0_2/4
  decat3/1(Out1) -> DDC0_3/1
  decat3/2(Out2) -> DDC0_3/2
  decat3/3(Out3) -> DDC0_3/3
  decat3/4(Out4) -> DDC0_3/4
  [sync_adc] -> DDC0_0/5
  [sync_adc] -> DDC0_1/5
  [sync_adc] -> DDC0_2/5
  [sync_adc] -> DDC0_3/5
  [fft_shift] -> fft/2
  [fft_shift] -> fft1/2
  DDC0_0/1 -> [ant1_pol1_ddc]
  DDC0_0/2 -> [sync_ant1_ddc]
  [sync_ant1_ddc] -> pfb_fir/1
  [ant1_pol1_ddc] -> pfb_fir/2
  [ant1_pol2_ddc] -> pfb_fir/3
  DDC0_1/1 -> [ant1_pol2_ddc]
  DDC0_2/1 -> [ant2_pol1_ddc]
  DDC0_2/2 -> [sync_ant2_ddc]
  DDC0_3/1 -> [ant2_pol2_ddc]
  [sync_ant2_ddc] -> pfb_fir1/1
  [ant2_pol1_ddc] -> pfb_fir1/2
  [ant2_pol2_ddc] -> pfb_fir1/3
  fft/1 -> [sync_ant1_fft]
  fft/2 -> [ant1_pol1_fft]
  fft/3 -> [ant1_pol2_fft]
  fft1/2 -> [ant2_pol1_fft]
  fft1/3 -> [ant2_pol2_fft]
  fft_tvg/2(sync_out) -> dbuf_ct_sram/2, [sync_presram]
  one_ant_a_time/1(dout) -> [ant12_pol12_reorder]
  [ant12_pol12_reorder] -> Concat10/2, Delay11/1
  one_ant_a_time/2(sync_out) -> [sync_reorder]
  [sync_reorder] -> Counter1/1, oob/1(sync)
  [ant12_pol12_rnd] -> fft_tvg/1(din)
  [sync_rnd] -> fft_tvg/2(sync)
  [xaui_ctrl_data] -> Mux2/2
  XAUI0/1(rx_data) -> Slice1/1, Slice2/1
  Register/1 -> [xaui_ctrl_data]
  Mux1/1 -> decat4/1(In1)
  decat4/1(Out1) -> calc_adc_sum_sq/1(In1)
  decat4/2(Out2) -> calc_adc_sum_sq/2(In2)
  decat4/3(Out3) -> calc_adc_sum_sq/3(In3)
  decat4/4(Out4) -> calc_adc_sum_sq/4(In4)
  calc_adc_sum_sq/1(sum_sq) -> adc_sum_sq/1
  Slice17/1 -> [input_sel]
  [input_sel] -> Mux1/1
  [ant1_pol1_adc] -> Mux1/2
  [ant1_pol2_adc] -> Mux1/3
  [ant2_pol1_adc] -> Mux1/4
  [ant2_pol2_adc] -> Mux1/5
  Delay1/1 -> Slice8/1, Slice7/1, Slice6/1, Slice3/1, Slice21/1, Slice17/1
  pfb_fir/2 -> downshift/1(din)
  downshift/1(dout) -> fft/3
  pfb_fir/3 -> downshift1/1(din)
  downshift1/1(dout) -> fft/4
  pfb_fir1/2 -> downshift2/1(din)
  downshift2/1(dout) -> fft1/3
  pfb_fir1/3 -> downshift3/1(din)
  downshift3/1(dout) -> fft1/4
  equalizer/1(dout) -> [ant12_pol12_rnd]
  equalizer/2(sync_out) -> [sync_rnd]
  [ant1_pol1_fft] -> equalizer/1(a1p1)
  [ant1_pol2_fft] -> equalizer/2(a1p2)
  [ant2_pol1_fft] -> equalizer/3(a2p1)
  [ant2_pol2_fft] -> equalizer/4(a2p2)
  [sync_ant1_fft] -> equalizer/5(sync)
  Slice1/1 -> Register/1
  [xaui_coeff] -> Mux7/2
  [xaui_coeff_en] -> Mux6/2
  Constant4/1 -> Mux6/3
  Constant5/1 -> eq_coeff/1
  eq_coeff/1 -> Mux7/3
  Slice20/1 -> Logical5/1
  Mux6/1 -> Logical5/2
  Mux7/1 -> Slice9/1, Slice22/1, Slice20/1
  Slice9/1 -> [coeff]
  Logical5/1 -> [coeff_en]
  [coeff] -> equalizer/6(coeff)
  [coeff_en] -> equalizer/7(coeff_we)
  [coeff_addr] -> equalizer/8(coeff_addr)
  Slice22/1 -> [coeff_addr]
  Delay2/1 -> fft/1
  Delay4/1 -> fft1/1
  XAUI0/4(rx_valid) -> Logical/1
  Inverter/1 -> Logical/2
  Logical/1 -> Delay/1, Register/2, Register1/2
  Slice2/1 -> Register1/1
  Register1/1 -> [xaui_coeff]
  neg_edge_ext/1(out) -> led_link_dn/1, Inverter/1
  clk_div_2/1 -> clk_out/1
  Delay/1 -> [xaui_coeff_en]
  Mux/1 -> XAUI0/4(tx_outofband)
  Constant/1 -> Mux/3
  oob/1(oob) -> Mux/2
  err_clear_sim5/1 -> oob_sel/1
  oob_sel/1 -> Slice18/1
  Slice18/1 -> Mux/1
  Constant3/1 -> XAUI1/1(rx_get)
  Constant6/1 -> XAUI1/2(rx_reset)
  Delay3/1 -> Concat1/1
  Concat1/1 -> XAUI1/3(tx_data)
  Counter2/1 -> Slice10/1, Slice4/1
  Slice10/1 -> XAUI1/5(tx_valid)
  Slice4/1 -> oob1/2(antbit)
  [mrst] -> oob1/3(mrst)
  [ant12_pol12_reorder] -> Concat1/2, Delay3/1
  [sync_reorder] -> Counter2/1, oob1/1(sync)
  Mux3/1 -> XAUI1/4(tx_outofband)
  Constant2/1 -> Mux3/3
  oob1/1(oob) -> Mux3/2
  err_clear_sim1/1 -> oob_sel1/1
  oob_sel1/1 -> Slice13/1
  Slice13/1 -> Mux3/1
  adc0/9 -> Logical1/1
  adc0/10 -> Logical1/2
  adc0/11 -> Logical1/3
  adc0/12 -> Logical1/4
  adc1/9 -> Logical2/1
  adc1/10 -> Logical2/2
  adc1/11 -> Logical2/3
  adc1/12 -> Logical2/4
  Logical1/1 -> [adc0_clip]
  Logical2/1 -> [adc1_clip]
  [adc0_clip] -> Logical6/1
  [adc1_clip] -> Logical6/2
  sync_gen/3(armed) -> led_arm/1
  Logical6/1 -> pulse_ext3/1(in)
  pulse_ext3/1(out) -> led_adc_clip/1
  pulse_ext4/1(out) -> led_eq_clip/1
  equalizer/3(clip) -> pulse_ext4/1(in)
